simulink model "ev-dab-sab-isolated-converter-model"  (R2025a)
settings: Solver=VariableStepAuto  StartTime=0.0  StopTime=5e-3  RelTol=1e-3
undefined symbols (not defined in the file): fsw, N, parallel_G
libraries: fl_lib x10, ee_lib x6, nesl_utility x5, simulink x1, slpidlib x1, spsSawtoothGeneratorLib x1
settings Model: VariantFading=off  Creator=cviana  LastModifiedBy=ahmed
settings RTWCC: GPUComputeCapability=3.5

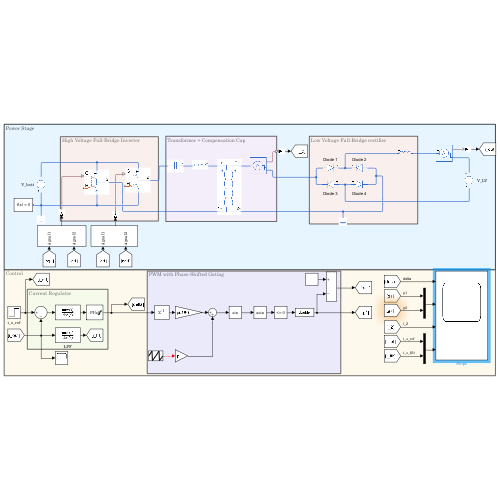
[thumbnail: Simulink's stored preview of the top-level diagram]
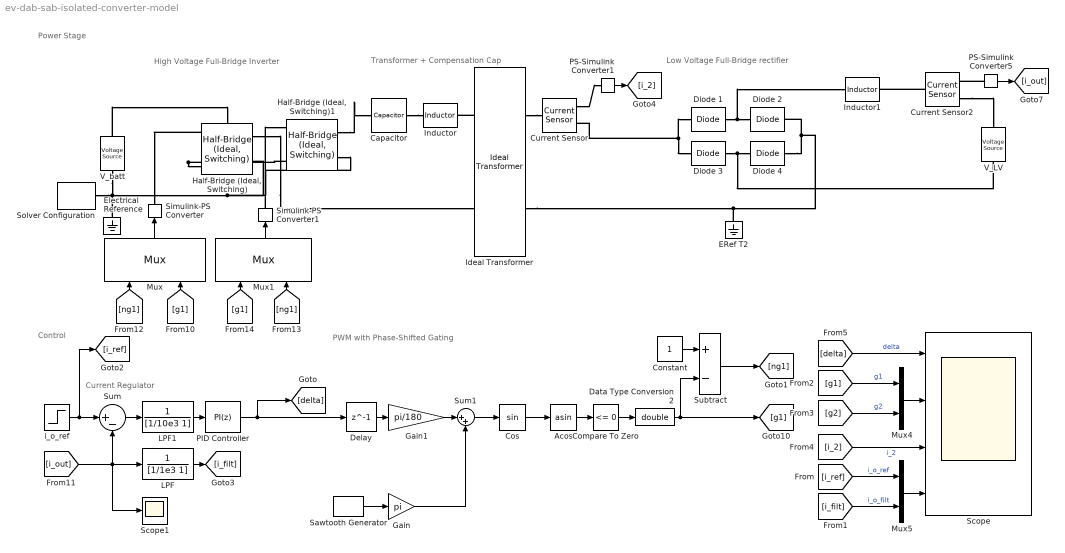
== system ev-dab-sab-isolated-converter-model ==
  note: Control
  note: Power Stage
  note: Transformer + Compensation Cap
  note: High Voltage Full-Bridge Inverter
  note: PWM with Phase-Shifted Gating
  note: Current Regulator
  note: Low Voltage Full-Bridge rectifier
  Acos : Trigonometry  Operator=asin
  Capacitor : fl_lib/Electrical/Electrical Elements/Capacitor  c=C F  r=1e-6 Ohm  g=parallel_G 1/Ohm  i_specify=off  i_priority=None  i=0 A  i_nominal_specify=off  i_nominal_value=1  i_nominal_unit=A  v_specify=off  v_priority=None  v=0 V  v_nominal_specify=off  v_nominal_value=1  v_nominal_unit=V  vc_specify=off  vc_priority=High  vc=0 V  vc_nominal_specify=off  vc_nominal_value=1  vc_nominal_unit=V
  Compare To Zero : simulink/Logic and Bit Operations/Compare To Zero  relop=<=  OutDataTypeStr=boolean
  Constant : Constant
  Cos : Trigonometry
  Current Sensor : fl_lib/Electrical/Electrical Sensors/Current Sensor
  Current Sensor2 : fl_lib/Electrical/Electrical Sensors/Current Sensor
  Data Type Conversion2 : DataTypeConversion  OutDataTypeStr=double  SaturateOnIntegerOverflow=off  RndMeth=Floor
  Delay : Delay  DelayLength=1  SampleTime=1/fsw
  Diode {1..4} (4 alike) : fl_lib/Electrical/Electrical Elements/Diode  Vf=0.6 V  Ron=0.3 Ohm  Goff=1e-08 1/Ohm  i_specify=off  i_priority=High  i=0 A  i_nominal_specify=off  i_nominal_value=1  i_nominal_unit=A  v_specify=off  v_priority=High  v=0 V  v_nominal_specify=off  v_nominal_value=1  v_nominal_unit=V
  ERef T2 : fl_lib/Electrical/Electrical Elements/Electrical Reference
  Electrical Reference : fl_lib/Electrical/Electrical Elements/Electrical Reference
  Gain : Gain  Gain=pi
  Gain1 : Gain  Gain=pi/180
  "Half-Bridge (Ideal, Switching)" : ee_lib/Semiconductors & Converters/Half-Bridge (Ideal, Switching)  control_port=ee.enum.controlport.ps  device_type=ee.enum.converters.switches.mosfet  gto_Vgt=6 V  gto_Vgt_off=-1 V  gto_Ih=1 A  gto_thermal_loss_option=ee.enum.converters.thermalLossOption.constantvalues  gto_Vf=0.8 V  gto_Ron=0.001 Ohm  gto_Von_data=[0, .1, .6, .8, 1, 1.3, 1.6, 2, 2.4; 0, .1, .7, 1, 1.2, 1.5, 1.9, 2.4, 2.8] V  gto_Tj=[298.15, 398.15] K  gto_Iout_data=[0, .1, 1, 5, 10, 20, 40, 70, 100] A  igbt_Vth=6 V  igbt_thermal_loss_option=ee.enum.converters.thermalLossOption.constantvalues  igbt_Vf=0.8 V  igbt_Ron=0.001 Ohm  igbt_Von_data=[0, .1, .6, .8, 1, 1.3, 1.6, 2, 2.4; 0, .1, .7, 1, 1.2, 1.5, 1.9, 2.4, 2.8] V  igbt_Tj=[298.15, 398.15] K  igbt_Iout_data=[0, .1, 1, 5, 10, 20, 40, 70, 100] A  mosfet_Vth=0.5 V  mosfet_thermal_loss_option=ee.enum.converters.thermalLossOption.constantvalues  mosfet_Rds=0.0001 Ohm  mosfet_Von_data=[0, 1.1, 1.3, 1.45, 1.75, 2.25, 2.7; 0, 1, 1.15, 1.35, 1.7, 2.35, 3] V  mosfet_Tj=[298.15, 398.15] K  mosfet_Iout_data=[0, 10, 50, 100, 200, 400, 600] A  Goff=1e-6 1/Ohm  gto_Eon_data=[0, .0024, .024, .12, .2, .48, 1.04, 2.16, 3.24; 0, .003, .03, .15, .25, .6, 1.3, 2.7, 4.05] * 1e-3 J  igbt_Eon_data=[0, .0024, .024, .12, .2, .48, 1.04, 2.16, 3.24; 0, .003, .03, .15, .25, .6, 1.3, 2.7, 4.05] * 1e-3 J  mosfet_Eon_data=[0, .29, 1.43, 2.86, 5.71, 13.14, 22.86; 0, .57, 2.63, 5.14, 10.29, 20.57, 30.29] * 1e-3 J  gto_Eoff_data=[0, .0007, .0066, .033, .066, .17, .33, .83, 1.5; 0, .001, .01, .05, .1, .25, .5, 1.2, 2.2] * 1e-3 J  igbt_Eoff_data=[0, .0007, .0066, .033, .066, .17, .33, .83, 1.5; 0, .001, .01, .05, .1, .25, .5, 1.2, 2.2] * 1e-3 J  mosfet_Eoff_data=[0, .21, 1.07, 2.14, 4.29, 9.86, 17.14; 0, .43, 1.97, 3.86, 7.71, 15.43, 22.71] * 1e-3 J  igbt_Eon_data_3D=[zeros(2, 9, 3)] J  mosfet_Eon_data_3D=[zeros(2, 7, 3)] J  igbt_Eoff_data_3D=[zeros(2, 9, 3)] J  mosfet_Eoff_data_3D=[zeros(2, 7, 3)] J  gto_Erec_data=[0, .0031, .021, .11, .21, .43, .99, 1.71, 3.078; 0, .0041, .043, .2, .39, .77, 1.54, 2.27, 4.08] * 1e-3 J  igbt_Erec_data=[0, .0031, .021, .11, .21, .43, .99, 1.71, 3.078; 0, .0041, .043, .2, .39, .77, 1.54, 2.27, 4.08] * 1e-3 J  mosfet_Erec_data=[0, .21, 1.23, 3.08, 7.64, 16.76, 25.88; 0, .39, 1.78, 4.08, 10.11, 22.18, 34.25] * 1e-3 J  gto_Tj_loss=[298.15, 398.15] K  igbt_Tj_loss=[298.15, 398.15] K  mosfet_Tj_loss=[298.15, 398.15] K  gto_Iout_data_loss=[0, .1, 1, 5, 10, 20, 40, 70, 100] A  igbt_Iout_data_loss=[0, .1, 1, 5, 10, 20, 40, 70, 100] A  mosfet_Iout_data_loss=[0, 10, 50, 100, 200, 400, 600] A  gto_Eon_scalar=22.86e-3 J  igbt_Eon_scalar=22.86e-3 J  mosfet_Eon_scalar=22.86e-3 J  gto_Eoff_scalar=17.14e-3 J  igbt_Eoff_scalar=17.14e-3 J  mosfet_Eoff_scalar=17.14e-3 J  gto_Erec_scalar=5.70e-3 J  igbt_Erec_scalar=5.70e-3 J  mosfet_Erec_scalar=5.70e-3 J  gto_Iout_scalar=600 A  igbt_Iout_scalar=600 A  mosfet_Iout_scalar=600 A  igbt_tabulateWithVce=false  mosfet_tabulateWithVds=false  igbt_Vce_loss=[0, 150, 300] V  mosfet_Vds_loss=[0, 150, 300] V  Voff=300 V  gto_Eoff_natural_commutation=10e-3 J  applySwLossToSupply=false  tauApplySwLoss=1e-3 s  diode_param=ee.enum.include.no  diode_ModelType=ee.enum.converters.diodeModelType.pwl  diode_TableType=ee.enum.diode.tableType.IfMat  diode_ReverseIVType=ee.enum.diode.diodeReverseIV.constant  diode_IfMat=[.07, .12, .19, 1.75, 4.24, 7.32, 11.2; .16, .3, .72, 2.14, 4.02, 6.35, 9.12] A  diode_VfMat=[.9, 1.15, 1.25, 1.5, 1.75, 2.17, 2.6, 2.85; .58, .68, .75, 1.1, 1.38, 1.77, 2.27, 2.7] V  diode_TjVec=[25, 125] degC  diode_VfVec=[.5, .7, .9, 1.3, 1.7, 2.1, 2.5] V  diode_IfVec=[.1, .2, .5, 1, 2, 4, 7, 10] A  diode_IrMat=[1e-06, 2e-06, 5e-06, 1e-05, 2.5e-05, 5e-05, .0001; 2e-06, 5e-06, 1e-05, 4e-05, 8e-05, .0002, .0005] A  diode_VrMat=[10, 100, 200, 250, 300, 325, 350; 10, 70, 160, 220, 270, 300, 320] V  diode_VrVec=[10, 20, 40, 50, 70, 80, 100] V  diode_IrVec=[1e-06, 2e-06, 5e-06, 1e-05, 2e-05, 5e-05, .0001] A  diode_Vf=0.8 V  diode_Ron=0.001 Ohm  diode_Goff=1e-5 1/Ohm  separateThermalPort=false  separateThermalPortsForDiodes=false  thermal_network_parameterization=ee.enum.thermalNetworkTopology.external  thermal_mass_parameterization=ee.enum.thermalNetwork.timeconstant  Rth=[.03, .2] K/W  Rth_Cauer=[.03, .1, .2] K/W  Rth_Foster=[.03, .2] K/W  thermal_mass=[3, 25] J/K  thermal_mass_Cauer=[3, 10, 25] J/K  thermal_mass_Foster=[33, 50] J/K  thermal_time_constant=[.1, 5] s  thermal_time_constant_Cauer=[.1, 1, 5] s  thermal_time_constant_Foster=[1, 10] s  thermal_mass_initial_temperatures=[25, 25] degC  thermal_mass_initial_temperatures_Cauer=[25, 25, 25] degC  junction_thermal_mass=0.1 J/K  Tvec_initial_Foster=[25, 25, 25, 25] degC  RthDiode=[.03, .2] K/W  RthCauerDiode=[.03, .1, .2] K/W  RthFosterDiode=[.03, .2] K/W  ThermalMassDiode=[3, 25] J/K  ThermalMassCauerDiode=[3, 10, 25] J/K  ThermalMassFosterDiode=[33, 50] J/K  ThermalTauDiode=[.1, 5] s  ThermalTauCauerDiode=[.1, 1, 5] s  ThermalTauFosterDiode=[1, 10] s  ThermalMassInitTempDiode=[25, 25] degC  ThermalMassInitTempCauerDiode=[25, 25, 25] degC  JunctionThermalMassDiode=0.1 J/K  TVecInitialFosterDiode=[25, 25, 25, 25] degC  junction_temperature_specify=off  junction_temperature_priority=None  junction_temperature=25 degC  junction_temperature_nominal_specify=off  junction_temperature_nominal_value=1  junction_temperature_nominal_unit=degC  upperSwitchTemp_specify=off  upperSwitchTemp_priority=None  upperSwitchTemp=25 degC  upperSwitchTemp_nominal_specify=off  upperSwitchTemp_nominal_value=1  upperSwitchTemp_nominal_unit=degC  lowerSwitchTemp_specify=off  lowerSwitchTemp_priority=None  lowerSwitchTemp=25 degC  lowerSwitchTemp_nominal_specify=off  lowerSwitchTemp_nominal_value=1  lowerSwitchTemp_nominal_unit=degC  upperDiodeTemp_specify=off  upperDiodeTemp_priority=None  upperDiodeTemp=25 degC  upperDiodeTemp_nominal_specify=off  upperDiodeTemp_nominal_value=1  upperDiodeTemp_nominal_unit=degC  lowerDiodeTemp_specify=off  lowerDiodeTemp_priority=None  lowerDiodeTemp=25 degC  lowerDiodeTemp_nominal_specify=off  lowerDiodeTemp_nominal_value=1  lowerDiodeTemp_nominal_unit=degC
      settings: InternalSimscapePortConfiguration="{\"Bottom\":[{\"id\":\"n\",\"label\":\"-\",\"type\":\"foundation.electrical.electrical\"}],\"Left\":[{\"id\":\"G\",\"label\":\"G\",\"type\":\"input\"},{\"id\":\"H\",\"label\":\"H\",\"type\":\"foundation.thermal.thermal\"}],\"Right\":[{\"id\":\"o\",\"label\":\"o\",\"type\":\"foundation.electrical.electrical\"}],\"Top\":[{\"id\":\"p\",\"label\":\"+\",\"type\":\"foundation.electrical.electrical\"}]}"
  "Half-Bridge (Ideal, Switching)1" : ee_lib/Semiconductors & Converters/Half-Bridge (Ideal, Switching)  control_port=ee.enum.controlport.ps  device_type=ee.enum.converters.switches.mosfet  gto_Vgt=6 V  gto_Vgt_off=-1 V  gto_Ih=1 A  gto_thermal_loss_option=ee.enum.converters.thermalLossOption.constantvalues  gto_Vf=0.8 V  gto_Ron=0.001 Ohm  gto_Von_data=[0, .1, .6, .8, 1, 1.3, 1.6, 2, 2.4; 0, .1, .7, 1, 1.2, 1.5, 1.9, 2.4, 2.8] V  gto_Tj=[298.15, 398.15] K  gto_Iout_data=[0, .1, 1, 5, 10, 20, 40, 70, 100] A  igbt_Vth=6 V  igbt_thermal_loss_option=ee.enum.converters.thermalLossOption.constantvalues  igbt_Vf=0.8 V  igbt_Ron=0.001 Ohm  igbt_Von_data=[0, .1, .6, .8, 1, 1.3, 1.6, 2, 2.4; 0, .1, .7, 1, 1.2, 1.5, 1.9, 2.4, 2.8] V  igbt_Tj=[298.15, 398.15] K  igbt_Iout_data=[0, .1, 1, 5, 10, 20, 40, 70, 100] A  mosfet_Vth=0.5 V  mosfet_thermal_loss_option=ee.enum.converters.thermalLossOption.constantvalues  mosfet_Rds=0.0001 Ohm  mosfet_Von_data=[0, 1.1, 1.3, 1.45, 1.75, 2.25, 2.7; 0, 1, 1.15, 1.35, 1.7, 2.35, 3] V  mosfet_Tj=[298.15, 398.15] K  mosfet_Iout_data=[0, 10, 50, 100, 200, 400, 600] A  Goff=1e-6 1/Ohm  gto_Eon_data=[0, .0024, .024, .12, .2, .48, 1.04, 2.16, 3.24; 0, .003, .03, .15, .25, .6, 1.3, 2.7, 4.05] * 1e-3 J  igbt_Eon_data=[0, .0024, .024, .12, .2, .48, 1.04, 2.16, 3.24; 0, .003, .03, .15, .25, .6, 1.3, 2.7, 4.05] * 1e-3 J  mosfet_Eon_data=[0, .29, 1.43, 2.86, 5.71, 13.14, 22.86; 0, .57, 2.63, 5.14, 10.29, 20.57, 30.29] * 1e-3 J  gto_Eoff_data=[0, .0007, .0066, .033, .066, .17, .33, .83, 1.5; 0, .001, .01, .05, .1, .25, .5, 1.2, 2.2] * 1e-3 J  igbt_Eoff_data=[0, .0007, .0066, .033, .066, .17, .33, .83, 1.5; 0, .001, .01, .05, .1, .25, .5, 1.2, 2.2] * 1e-3 J  mosfet_Eoff_data=[0, .21, 1.07, 2.14, 4.29, 9.86, 17.14; 0, .43, 1.97, 3.86, 7.71, 15.43, 22.71] * 1e-3 J  igbt_Eon_data_3D=[zeros(2, 9, 3)] J  mosfet_Eon_data_3D=[zeros(2, 7, 3)] J  igbt_Eoff_data_3D=[zeros(2, 9, 3)] J  mosfet_Eoff_data_3D=[zeros(2, 7, 3)] J  gto_Erec_data=[0, .0031, .021, .11, .21, .43, .99, 1.71, 3.078; 0, .0041, .043, .2, .39, .77, 1.54, 2.27, 4.08] * 1e-3 J  igbt_Erec_data=[0, .0031, .021, .11, .21, .43, .99, 1.71, 3.078; 0, .0041, .043, .2, .39, .77, 1.54, 2.27, 4.08] * 1e-3 J  mosfet_Erec_data=[0, .21, 1.23, 3.08, 7.64, 16.76, 25.88; 0, .39, 1.78, 4.08, 10.11, 22.18, 34.25] * 1e-3 J  gto_Tj_loss=[298.15, 398.15] K  igbt_Tj_loss=[298.15, 398.15] K  mosfet_Tj_loss=[298.15, 398.15] K  gto_Iout_data_loss=[0, .1, 1, 5, 10, 20, 40, 70, 100] A  igbt_Iout_data_loss=[0, .1, 1, 5, 10, 20, 40, 70, 100] A  mosfet_Iout_data_loss=[0, 10, 50, 100, 200, 400, 600] A  gto_Eon_scalar=22.86e-3 J  igbt_Eon_scalar=22.86e-3 J  mosfet_Eon_scalar=22.86e-3 J  gto_Eoff_scalar=17.14e-3 J  igbt_Eoff_scalar=17.14e-3 J  mosfet_Eoff_scalar=17.14e-3 J  gto_Erec_scalar=5.70e-3 J  igbt_Erec_scalar=5.70e-3 J  mosfet_Erec_scalar=5.70e-3 J  gto_Iout_scalar=600 A  igbt_Iout_scalar=600 A  mosfet_Iout_scalar=600 A  igbt_tabulateWithVce=false  mosfet_tabulateWithVds=false  igbt_Vce_loss=[0, 150, 300] V  mosfet_Vds_loss=[0, 150, 300] V  Voff=300 V  gto_Eoff_natural_commutation=10e-3 J  applySwLossToSupply=false  tauApplySwLoss=1e-3 s  diode_param=ee.enum.include.no  diode_ModelType=ee.enum.converters.diodeModelType.pwl  diode_TableType=ee.enum.diode.tableType.IfMat  diode_ReverseIVType=ee.enum.diode.diodeReverseIV.constant  diode_IfMat=[.07, .12, .19, 1.75, 4.24, 7.32, 11.2; .16, .3, .72, 2.14, 4.02, 6.35, 9.12] A  diode_VfMat=[.9, 1.15, 1.25, 1.5, 1.75, 2.17, 2.6, 2.85; .58, .68, .75, 1.1, 1.38, 1.77, 2.27, 2.7] V  diode_TjVec=[25, 125] degC  diode_VfVec=[.5, .7, .9, 1.3, 1.7, 2.1, 2.5] V  diode_IfVec=[.1, .2, .5, 1, 2, 4, 7, 10] A  diode_IrMat=[1e-06, 2e-06, 5e-06, 1e-05, 2.5e-05, 5e-05, .0001; 2e-06, 5e-06, 1e-05, 4e-05, 8e-05, .0002, .0005] A  diode_VrMat=[10, 100, 200, 250, 300, 325, 350; 10, 70, 160, 220, 270, 300, 320] V  diode_VrVec=[10, 20, 40, 50, 70, 80, 100] V  diode_IrVec=[1e-06, 2e-06, 5e-06, 1e-05, 2e-05, 5e-05, .0001] A  diode_Vf=0.8 V  diode_Ron=0.001 Ohm  diode_Goff=1e-5 1/Ohm  separateThermalPort=false  separateThermalPortsForDiodes=false  thermal_network_parameterization=ee.enum.thermalNetworkTopology.external  thermal_mass_parameterization=ee.enum.thermalNetwork.timeconstant  Rth=[.03, .2] K/W  Rth_Cauer=[.03, .1, .2] K/W  Rth_Foster=[.03, .2] K/W  thermal_mass=[3, 25] J/K  thermal_mass_Cauer=[3, 10, 25] J/K  thermal_mass_Foster=[33, 50] J/K  thermal_time_constant=[.1, 5] s  thermal_time_constant_Cauer=[.1, 1, 5] s  thermal_time_constant_Foster=[1, 10] s  thermal_mass_initial_temperatures=[25, 25] degC  thermal_mass_initial_temperatures_Cauer=[25, 25, 25] degC  junction_thermal_mass=0.1 J/K  Tvec_initial_Foster=[25, 25, 25, 25] degC  RthDiode=[.03, .2] K/W  RthCauerDiode=[.03, .1, .2] K/W  RthFosterDiode=[.03, .2] K/W  ThermalMassDiode=[3, 25] J/K  ThermalMassCauerDiode=[3, 10, 25] J/K  ThermalMassFosterDiode=[33, 50] J/K  ThermalTauDiode=[.1, 5] s  ThermalTauCauerDiode=[.1, 1, 5] s  ThermalTauFosterDiode=[1, 10] s  ThermalMassInitTempDiode=[25, 25] degC  ThermalMassInitTempCauerDiode=[25, 25, 25] degC  JunctionThermalMassDiode=0.1 J/K  TVecInitialFosterDiode=[25, 25, 25, 25] degC  junction_temperature_specify=off  junction_temperature_priority=None  junction_temperature=25 degC  junction_temperature_nominal_specify=off  junction_temperature_nominal_value=1  junction_temperature_nominal_unit=degC  upperSwitchTemp_specify=off  upperSwitchTemp_priority=None  upperSwitchTemp=25 degC  upperSwitchTemp_nominal_specify=off  upperSwitchTemp_nominal_value=1  upperSwitchTemp_nominal_unit=degC  lowerSwitchTemp_specify=off  lowerSwitchTemp_priority=None  lowerSwitchTemp=25 degC  lowerSwitchTemp_nominal_specify=off  lowerSwitchTemp_nominal_value=1  lowerSwitchTemp_nominal_unit=degC  upperDiodeTemp_specify=off  upperDiodeTemp_priority=None  upperDiodeTemp=25 degC  upperDiodeTemp_nominal_specify=off  upperDiodeTemp_nominal_value=1  upperDiodeTemp_nominal_unit=degC  lowerDiodeTemp_specify=off  lowerDiodeTemp_priority=None  lowerDiodeTemp=25 degC  lowerDiodeTemp_nominal_specify=off  lowerDiodeTemp_nominal_value=1  lowerDiodeTemp_nominal_unit=degC
      settings: InternalSimscapePortConfiguration="{\"Bottom\":[{\"id\":\"n\",\"label\":\"-\",\"type\":\"foundation.electrical.electrical\"}],\"Left\":[{\"id\":\"G\",\"label\":\"G\",\"type\":\"input\"},{\"id\":\"H\",\"label\":\"H\",\"type\":\"foundation.thermal.thermal\"}],\"Right\":[{\"id\":\"o\",\"label\":\"o\",\"type\":\"foundation.electrical.electrical\"}],\"Top\":[{\"id\":\"p\",\"label\":\"+\",\"type\":\"foundation.electrical.electrical\"}]}"
  Ideal Transformer : fl_lib/Electrical/Electrical Elements/Ideal Transformer  n=1/N  i1_specify=off  i1_priority=None  i1=0 A  i1_nominal_specify=off  i1_nominal_value=1  i1_nominal_unit=A  v1_specify=off  v1_priority=None  v1=0 V  v1_nominal_specify=off  v1_nominal_value=1  v1_nominal_unit=V  i2_specify=off  i2_priority=None  i2=0 A  i2_nominal_specify=off  i2_nominal_value=1  i2_nominal_unit=A  v2_specify=off  v2_priority=None  v2=0 V  v2_nominal_specify=off  v2_nominal_value=1  v2_nominal_unit=V
  Inductor : ee_lib/Passive/Inductor  l=L H  enable_L_tol=ee.enum.toleranceApplication.none  L_tol=20  tol_distribution=ee.enum.toleranceDistribution.uniform  nSigma=4  r=10e-3 Ohm  g=1e-9 1/Ohm  enable_operating_limits=ee.enum.enable.no  operating_limit_action=ee.enum.passive.reportOpLim.warn  max_working_current=1 A  power_rating=1 W  i_L_specify=off  i_L_priority=High  i_L=0 A  i_L_nominal_specify=off  i_L_nominal_value=1  i_L_nominal_unit=A
  Inductor1 : ee_lib/Passive/Inductor  l=2e-6 H  enable_L_tol=ee.enum.toleranceApplication.none  L_tol=20  tol_distribution=ee.enum.toleranceDistribution.uniform  nSigma=4  r=0.12 Ohm  g=1e-9 1/Ohm  enable_operating_limits=ee.enum.enable.no  operating_limit_action=ee.enum.passive.reportOpLim.warn  max_working_current=1 A  power_rating=1 W  i_L_specify=off  i_L_priority=High  i_L=0 A  i_L_nominal_specify=off  i_L_nominal_value=1  i_L_nominal_unit=A
  LPF : TransferFcn  Denominator=[1/1e3 1]
  LPF1 : TransferFcn  Denominator=[1/10e3 1]
  Mux{,1,4..5} (4 alike) : Mux  Inputs=2
      Mux settings: DisplayOption=signals
      Mux1 settings: DisplayOption=signals
  PID Controller : slpidlib/PID Controller  Controller=PI  Form=Parallel  TimeDomain=Discrete-time  UseExternalTs=off  SampleTime=-1  IntegratorMethod=Forward Euler  FilterMethod=Forward Euler  ControllerParametersSource=internal  P=1  I=15000  UseKiTs=off  D=0  UseExternalDerivativeSource=off  N=100  UseFilter=on  TunerSelectOption=Transfer Function Based (PID Tuner App)  InitialConditionSource=internal  InitialConditionForIntegrator=0  InitialConditionForFilter=0  DifferentiatorICPrevScaledInput=0  ExternalReset=none  TrackingMode=off  Kt=1  LimitOutput=on  SatLimitsSource=internal  UpperSaturationLimit=90  LowerSaturationLimit=-90  LinearizeAsGain=on  AntiWindupMode=clamping  Kb=1  LimitIntegrator=off  UpperIntegratorSaturationLimit=inf  LowerIntegratorSaturationLimit=-inf  POutMin=[]  POutMax=[]  IOutMin=[]  IOutMax=[]  DOutMin=[]  DOutMax=[]  NOutMin=[]  NOutMax=[]  SumOutMin=[]  SumOutMax=[]  SaturationOutMin=[]  SaturationOutMax=[]  PParamMin=[]  PParamMax=[]  IParamMin=[]  IParamMax=[]  DParamMin=[]  DParamMax=[]  NParamMin=[]  NParamMax=[]  KbParamMin=[]  KbParamMax=[]  KtParamMin=[]  KtParamMax=[]  KbOutMin=[]  KbOutMax=[]  KtOutMin=[]  KtOutMax=[]  IntegratorOutMin=[]  IntegratorOutMax=[]  FilterOutMin=[]  FilterOutMax=[]  SumI1OutMin=[]  SumI1OutMax=[]  SumI2OutMin=[]  SumI2OutMax=[]  SumI3OutMin=[]  SumI3OutMax=[]  SumI4OutMin=[]  SumI4OutMax=[]  SumDOutMin=[]  SumDOutMax=[]  DifferentiatorOutMin=[]  DifferentiatorOutMax=[]  FilterDiffOutCoefMin=[]  FilterDiffOutCoefMax=[]  ReciprocalOutMin=[]  ReciprocalOutMax=[]  SumDenOutMin=[]  SumDenOutMax=[]  SumNumOutMin=[]  SumNumOutMax=[]  DivideOutMin=[]  DivideOutMax=[]  UdiffTsProdOutMin=[]  UdiffTsProdOutMax=[]  NTsProdOutMin=[]  NTsProdOutMax=[]  UintegralTsProdOutMin=[]  UintegralTsProdOutMax=[]  UngainTsProdOutMin=[]  UngainTsProdOutMax=[]  ClampingZeroOutDataTypeStr=Inherit: Inherit via back propagation  ClampingZeroOutMin=[]  ClampingZeroOutMax=[]  FilterDenConstantOutDataTypeStr=Inherit: Inherit via back propagation  FilterDenConstantOutMin=[]  FilterDenConstantOutMax=[]  PCopyOutDataTypeStr=Inherit: Inherit via back propagation  PCopyOutMin=[]  PCopyOutMax=[]  NCopyOutDataTypeStr=Inherit: Inherit via back propagation  NCopyOutMin=[]  NCopyOutMax=[]  IntegratorContinuousStateAttributes=''  IntegratorStateMustResolveToSignalObject=off  IntegratorRTWStateStorageClass=Auto  FilterContinuousStateAttributes=''  FilterStateMustResolveToSignalObject=off  FilterRTWStateStorageClass=Auto  ParallelPVariant=InternalParameters  IdealPVariant=Disabled  IVariant=InternalParameters  DVariant=Disabled  IntegratorVariant=Discrete  SatVariant=Enabled  AWVariant=DiscClampingParallel  PCopyVariant=Disabled  TRVariant=Disabled  FdbkBlocksVariant=Forward  IdealPFdbkVariant=Disabled  SatFdbkVariant=Disabled  DerivativeFilterVariant=Disabled  NVariant=Disabled  NCopyVariant=Disabled_SignalSpec  FilterICVariant=Disabled  IntegratorICVariant=InternalICs  ExternalResetVariant=Disabled  TRSumVariant=Passthrough  SumFdbkVariant=Disabled  SumVariant=Sum_PI  TsampFilterVariant=InternalTs  TsampNgainVariant=Passthrough  TsampIntegralVariant=Disabled_SignalSpec  ExternalSaturationOutDataTypeStr=Inherit: Same as second input  DerivativeSourceVariant=Disabled  PreIntVariant=InternalPreInt
  PS-Simulink Converter1 : nesl_utility/PS-Simulink Converter  PhysicalDomain=network_engine_domain  SubClassName=ps_output  LeftPortType=input  RightPortType=output  PseudoPeriodic=off  Frequencies=[]  VectorFormat=inherit  Unit=inherit  AffineConversion=off
  PS-Simulink Converter5 : nesl_utility/PS-Simulink Converter  PhysicalDomain=network_engine_domain  SubClassName=ps_output  LeftPortType=input  RightPortType=output  PseudoPeriodic=off  Frequencies=[]  VectorFormat=inherit  Unit=inherit  AffineConversion=off
  Sawtooth Generator : spsSawtoothGeneratorLib/Sawtooth Generator  Freq=fsw  Phase=180  Ts=0
  Scope : Scope  NumInputPorts=4
      settings: ActiveDisplayYMinimum=-107.83112420914549  ActiveDisplayYMaximum=70.480117882309429
  Scope1 : Scope
      settings: ActiveDisplayYMinimum=-163.74694  ActiveDisplayYMaximum=222.11926
  Simulink-PS Converter : nesl_utility/Simulink-PS Converter  PhysicalDomain=network_engine_domain  SubClassName=ps_input  LeftPortType=input  RightPortType=output  PseudoPeriodic=off  Frequencies=[]  NoiseDistribution=none  NoiseParameters=[]  Unit=1  AffineConversion=off  FilteringAndDerivatives=provide  SimscapeFilterOrder=1  InputFilterTimeConstant=0.001  UdotUserProvided=0
  Simulink-PS Converter1 : nesl_utility/Simulink-PS Converter  PhysicalDomain=network_engine_domain  SubClassName=ps_input  LeftPortType=input  RightPortType=output  PseudoPeriodic=off  Frequencies=[]  NoiseDistribution=none  NoiseParameters=[]  Unit=1  AffineConversion=off  FilteringAndDerivatives=provide  SimscapeFilterOrder=1  InputFilterTimeConstant=0.001  UdotUserProvided=0
  Solver Configuration : nesl_utility/Solver Configuration  PhysicalDomain=network_engine_domain  SubClassName=solver  LeftPortType=input  RightPortType=generic  Tones=[]  Harmonics=[]  SimulateNoise=off  Profile=off  UseLocalSampling=off  EnableSwitchedLinearOptims=on  FrequencyDomain=off  UseCCode=off  RelTol=0.001  AbsTol=0.001  MinStep=1e-09  ToWorkspace=off  RevertToSquareIcSolve=off  NumHomotopyIterations=100  PhasorMode=off  PhasorModeNumHarmonics=1  ConsistencySolver=NEWTON_XTOL_AFTER_FTOL  IndexReductionMethod=DerivativeReplacement  DoDC=off  ResidualTolerance=1e-09  ConsistencyTolSource=GLOBAL  ConsistencyAbsTol=0.001  ConsistencyRelTol=0.001  ConsistencyTolFactor=0.001  UseLocalSolver=off  LocalSolverChoice=NE_BACKWARD_EULER_ADVANCER  ResolveIndetEquations=on  FunctionEvalNumThread=1  LocalSolverSampleTime=0.001  DoFixedCost=off  MaxNonlinIter=3  MaxModeIter=2  ComputeImpulses=off  ImpulseIterations=2  LinearAlgebra=auto  LinearAlgebraNumThread=0  EquationFormulation=NE_TIME_EF  DelaysMemoryBudget=1024  AutomaticFiltering=on  FilteringTimeConstant=0.001  PartitionStorageMethod=AS_NEEDED  PartitionMemoryBudget=1024  PartitionMethod=ROBUST  MultibodyUseLocalSolver=off  MultibodyLocalSolverChoice=ODE1  MultibodyLocalSolverSampleTime=0.001
  Subtract : Sum  Inputs=+-
  Sum : Sum  Inputs=|+-
  Sum1 : Sum  Inputs=|++
  V_LV : ee_lib/Sources/Voltage Source  dc_voltage=12 V  ac_voltage=0 V  ac_shift=0 rad  ac_frequency=60 Hz  noise_mode=ee.enum.sources.noise.Disabled  PSD=0 V^2/Hz  sample_time=1e-3 s  repeatability=ee.enum.sources.repeatability.NotRepeatable  user_seed=0  auto_seed=977810714  i_specify=off  i_priority=None  i=0 A  i_nominal_specify=off  i_nominal_value=1  i_nominal_unit=A  v_specify=off  v_priority=None  v=0 V  v_nominal_specify=off  v_nominal_value=1  v_nominal_unit=V
  V_batt : ee_lib/Sources/Voltage Source  dc_voltage=3000 V  ac_voltage=0 V  ac_shift=0 rad  ac_frequency=60 Hz  noise_mode=ee.enum.sources.noise.Disabled  PSD=0 V^2/Hz  sample_time=1e-3 s  repeatability=ee.enum.sources.repeatability.NotRepeatable  user_seed=0  auto_seed=3499211588  i_specify=off  i_priority=None  i=0 A  i_nominal_specify=off  i_nominal_value=1  i_nominal_unit=A  v_specify=off  v_priority=None  v=0 V  v_nominal_specify=off  v_nominal_value=1  v_nominal_unit=V
  i_o_ref : Step  Time=50/fsw  After=100  SampleTime=0
  wires:
  i_o_ref/1 -> [i_ref], Sum/1
  LPF/1 -> [i_filt]
  Acos/1 -> Compare To Zero/1
  Compare To Zero/1 -> Data Type Conversion2/1
  Sawtooth Generator/1 -> Gain/1
  Sum1/1 -> Cos/1
  Gain1/1 -> Sum1/1
  Gain/1 -> Sum1/2
  Cos/1 -> Acos/1
  [ng1] -> Mux1/2
  Mux1/1 -> Simulink-PS Converter1/1
  Subtract/1 -> [ng1]
  [g1] -> Mux/2
  [g1] -> Mux1/1
  [ng1] -> Mux/1
  Constant/1 -> Subtract/1
  Data Type Conversion2/1 -> Subtract/2, [g1]
  Mux/1 -> Simulink-PS Converter/1
  [g1] -> Mux4/1  "g1"
  [g2] -> Mux4/2  "g2"
  [i_filt] -> Mux5/2  "i_o_filt"
  [i_ref] -> Mux5/1  "i_o_ref"
  [i_out] -> Scope1/1, Sum/2, LPF/1
  Sum/1 -> LPF1/1
  LPF1/1 -> PID Controller/1
  PID Controller/1 -> Delay/1, [delta]
  PS-Simulink Converter1/1 -> [i_2]
  Mux5/1 -> Scope/4
  Delay/1 -> Gain1/1
  [i_2] -> Scope/3  "i_2"
  [delta] -> Scope/1  "delta"
  Mux4/1 -> Scope/2
  PS-Simulink Converter5/1 -> [i_out]
  connections:
  Ideal Transformer/LConn1 -- Inductor/RConn1
  "Half-Bridge (Ideal, Switching)1"/LConn3 -- V_batt/LConn1 -- "Half-Bridge (Ideal, Switching)"/LConn3
  V_batt/RConn1 -- Electrical Reference/LConn1 -- Solver Configuration/RConn1 -- "Half-Bridge (Ideal, Switching)1"/RConn2 -- "Half-Bridge (Ideal, Switching)"/RConn2
  "Half-Bridge (Ideal, Switching)"/LConn1 -- Simulink-PS Converter/RConn1
  Simulink-PS Converter1/RConn1 -- "Half-Bridge (Ideal, Switching)1"/LConn1
  Capacitor/RConn1 -- Inductor/LConn1
  "Half-Bridge (Ideal, Switching)1"/RConn1 -- Capacitor/LConn1
  "Half-Bridge (Ideal, Switching)"/RConn1 -- Ideal Transformer/LConn2
  Ideal Transformer/RConn1 -- Current Sensor/LConn1
  Current Sensor/RConn1 -- PS-Simulink Converter1/LConn1
  Diode 4/RConn1 -- ERef T2/LConn1 -- Ideal Transformer/RConn2 -- Diode 2/LConn1
  Diode 3/RConn1 -- Diode 1/LConn1 -- Current Sensor/RConn2
  Diode 3/LConn1 -- Diode 4/LConn1 -- V_LV/RConn1
  PS-Simulink Converter5/LConn1 -- Current Sensor2/RConn1
  Current Sensor2/RConn2 -- V_LV/LConn1
  Diode 1/RConn1 -- Inductor1/LConn1 -- Diode 2/RConn1
  Current Sensor2/LConn1 -- Inductor1/RConn1
